simulink model "clik_phi_inverse"  (Simulink 10.2)
settings: Solver=ode1  StartTime=0.0  StopTime=4  FixedStep=0.001  RelTol=1e-3
undefined symbols (not defined in the file or in its folder): DiscIntNeverNeededParam, q0, Tc
settings Model: Creator=Xp  LastModifiedBy=Megha
settings DataIOCC: LimitDataPoints=on
settings OptimizationCC: ExpressionDepthLimit=2147483647  InitFltsAndDblsToZero=on
settings DebuggingCC: SaveWithParameterizedLinksMsg=none  SolverPrmCheckMsg=warning  MultiTaskDSMMsg=warning  MultiTaskCondExecSysMsg=none  StateNameClashWarn=warning
settings SFSimCC: SimUseLocalCustomCode=on
settings RTWCC: RTWUseLocalCustomCode=on
settings ConfigComp: CovExternalEMLEnable=on

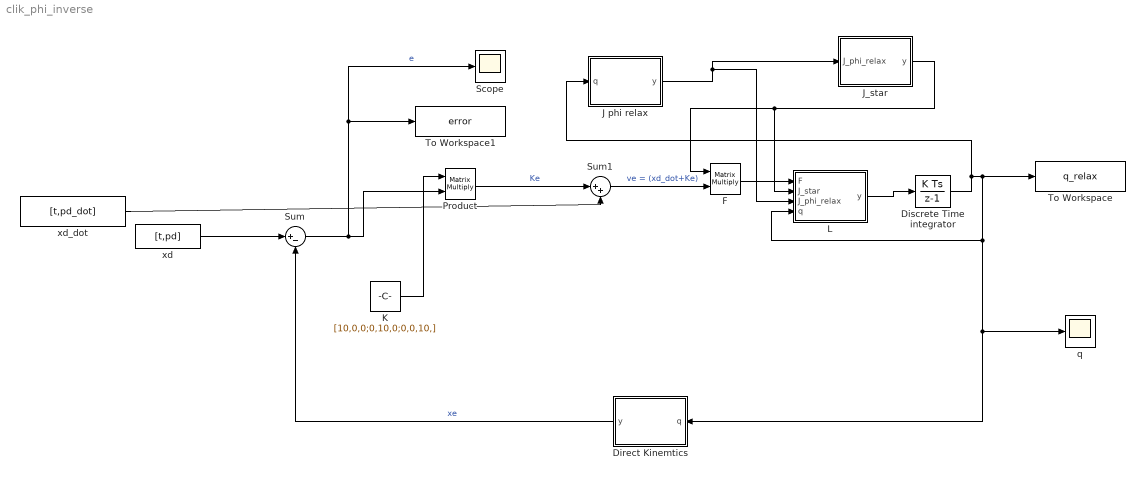
== system clik_phi_inverse ==
  Direct Kinemtics : MATLAB Function  TreatAsAtomicUnit=on
  Discrete Time integrator : DiscreteIntegrator  InitialCondition=q0  SampleTime=Tc  ICPrevOutput=DiscIntNeverNeededParam  ICPrevScaledInput=DiscIntNeverNeededParam
  F : Product  Multiplication=Matrix(*)
  J phi relax : MATLAB Function  TreatAsAtomicUnit=on
  J_star : MATLAB Function  TreatAsAtomicUnit=on
  K : Constant  Value=[10,0,0;0,10,0;0,0,10,]
  L : MATLAB Function  TreatAsAtomicUnit=on
  Product : Product  Multiplication=Matrix(*)
  Scope : Scope
  Sum : Sum  Inputs=|+-
  Sum1 : Sum  Inputs=|++
  To Workspace : ToWorkspace  VariableName=q_relax  SaveFormat=Timeseries  SampleTime=-1
  To Workspace1 : ToWorkspace  VariableName=error  SaveFormat=Timeseries  SampleTime=-1
  q : Scope
  xd : FromWorkspace  VariableName=[t,pd]
  xd_dot : FromWorkspace  VariableName=[t,pd_dot]
  wires:
  Direct Kinemtics/1(y) -> Sum/2  "xe"
  Product/1 -> Sum1/1  "Ke"
  Sum/1 -> To Workspace1/1, Scope/1, Product/2  "e"
  K/1 -> Product/1
  xd/1 -> Sum/1
  xd_dot/1 -> Sum1/2
  J_star/1(y) -> F/1, L/2(J_star)
  J phi relax/1(y) -> J_star/1(J_phi_relax), L/3(J_phi_relax)
  Discrete Time integrator/1 -> J phi relax/1(q), L/4(q), q/1, Direct Kinemtics/1(q), To Workspace/1
  F/1 -> L/1(F)
  L/1(y) -> Discrete Time integrator/1
  Sum1/1 -> F/2  "ve = (xd_dot+Ke)"

== matlab function J_star ==
  data: J_phi_relax input double; y output double
function y = fcn(J_phi_relax)
J_star = J_phi_relax.' * (inv((J_phi_relax*J_phi_relax.')));
y = J_star;

== matlab function J phi relax ==
  data: q input double; y output double
function y = fcn(q)
theta_1 = q(1);
theta_2 = q(2);
d3 = q(3);
theta_4 = q(4);
j1 =[- sin(theta_1)/2 - (cos(theta_1)*sin(theta_2))/2 - (cos(theta_2)*sin(theta_1))/2, - (cos(theta_1)*sin(theta_2))/2 - (cos(theta_2)*sin(theta_1))/2, 0, 0];
j2 = [  cos(theta_1)/2 + (cos(theta_1)*cos(theta_2))/2 - (sin(theta_1)*sin(theta_2))/2,   (cos(theta_1)*cos(theta_2))/2 - (sin(theta_1)*sin(theta_2))/2, 0, 0];
j3 = [0,0,-1, 0];
J_phi_relax  = [j1;j2;j3];
y = J_phi_relax;

== matlab function Direct Kinemtics ==
  data: q input double; y output double
function y = fcn(q)
q
theta_1 = q(1);
theta_2 = q(2);
d3 = q(3);
theta_4 = q(4);
t14 = cos(theta_1)/2 + (cos(theta_1)*cos(theta_2))/2 - (sin(theta_1)*sin(theta_2))/2;
t24 = sin(theta_1)/2 + (cos(theta_1)*sin(theta_2))/2 + (cos(theta_2)*sin(theta_1))/2;
t34 = 1-d3;
pe = [t14;t24;t34];
xe =[pe];
y = xe;

== matlab function L ==
  data: F input double; y output double; J_star input double; J_phi_relax input double; q input double
function y = fcn(F,J_star,J_phi_relax,q)
theta_1 = q(1);
theta_2 = q(2);
d3 = q(3);
theta_4 = q(4);
k0 = 10000*eye(4,4);
q0_dot= k0 * [ (-1/(4*pi*pi))*theta_1 ; (-4/(9*pi*pi))*( theta_2+(pi/8) ) ; (-4/9)*( d3-0.625 ) ; (-1/(64*pi*pi))*theta_4 ];
I_n = eye(4,4)
q_dot = F + [I_n - J_star * J_phi_relax]*q0_dot
y = q_dot;
